simulink model "ct_sfun_sf_control"  (R2015a)
settings: Solver=ode45  StartTime=0.0  StopTime=10  RelTol=1e-3
settings Model: Creator=Arnab Banerjee  LastModifiedBy=Arnab Banerjee

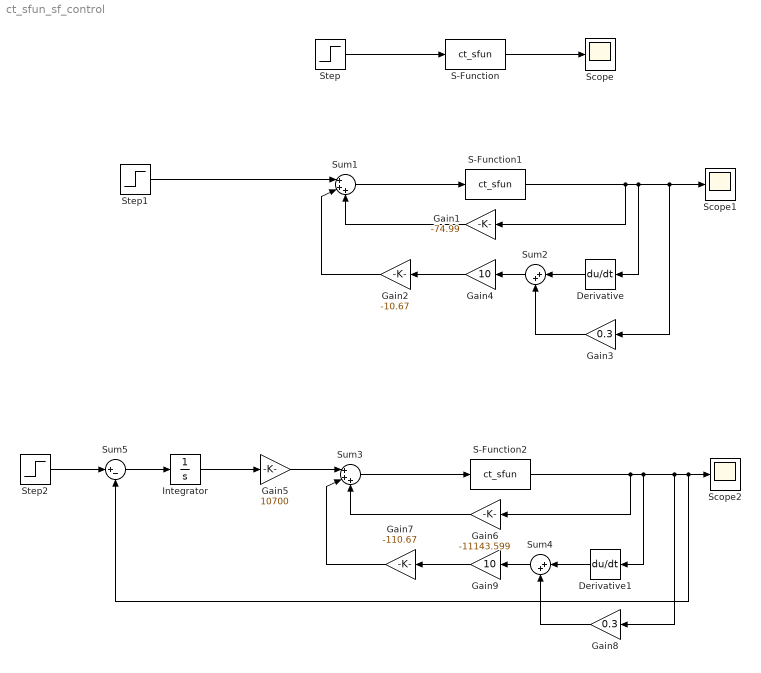
== system ct_sfun_sf_control ==
  Derivative : Derivative
  Derivative1 : Derivative
  Gain1 : Gain  Gain=-74.99
  Gain2 : Gain  Gain=-10.67
  Gain3 : Gain  Gain=0.3
  Gain4 : Gain  Gain=10
  Gain5 : Gain  Gain=10700
  Gain6 : Gain  Gain=-11143.599
  Gain7 : Gain  Gain=-110.67
  Gain8 : Gain  Gain=0.3
  Gain9 : Gain  Gain=10
  Integrator : Integrator
  S-Function : S-Function  FunctionName=ct_sfun
  S-Function1 : S-Function  FunctionName=ct_sfun
  S-Function2 : S-Function  FunctionName=ct_sfun
  Scope : Scope
  Scope1 : Scope
  Scope2 : Scope
      settings: SaveName=ScopeData2
  Step : Step  Time=0  SampleTime=0
  Step1 : Step  Time=0  SampleTime=0
  Step2 : Step  Time=0  SampleTime=0
  Sum1 : Sum  Inputs=|+++
  Sum2 : Sum  Inputs=|++
  Sum3 : Sum  Inputs=|+++
  Sum4 : Sum  Inputs=|++
  Sum5 : Sum  Inputs=|+-
  wires:
  S-Function/1 -> Scope/1
  Step/1 -> S-Function/1
  S-Function1/1 -> Gain1/1, Derivative/1, Gain3/1, Scope1/1
  Sum1/1 -> S-Function1/1
  Gain1/1 -> Sum1/3
  Gain2/1 -> Sum1/2
  Step1/1 -> Sum1/1
  Sum2/1 -> Gain4/1
  Derivative/1 -> Sum2/1
  Gain3/1 -> Sum2/2
  Gain4/1 -> Gain2/1
  S-Function2/1 -> Gain6/1, Derivative1/1, Gain8/1, Sum5/2, Scope2/1
  Sum3/1 -> S-Function2/1
  Gain6/1 -> Sum3/3
  Gain7/1 -> Sum3/2
  Sum4/1 -> Gain9/1
  Derivative1/1 -> Sum4/1
  Gain8/1 -> Sum4/2
  Gain9/1 -> Gain7/1
  Gain5/1 -> Sum3/1
  Integrator/1 -> Gain5/1
  Step2/1 -> Sum5/1
  Sum5/1 -> Integrator/1
